simulink model "RightInvariant_EKF"  (R2016b)
settings: Solver=FixedStepDiscrete  StartTime=0.0  StopTime=inf  RelTol=1e-3  EnableMultiTasking=on
InitFcn:
  | RIEKF_InitFcn;
libraries: StateEstimation x3, dspfdesign x2, slrtlib x1, UDP_Communication x1
settings Model: xpc_rtwmakecfg_data=_xpcethercatlib_  ParamWorkspaceSource=ReferencedWorkspace  Creator=robot  LastModifiedBy=Ross Hartley
settings SolverCC: EnableConcurrentExecution=on  ConcurrentTasks=on
settings DataIOCC: SaveFormat=Array  SaveOutput=off  SignalLogging=off  DSMLogging=off  VisualizeSimOutput=off  SaveTime=off
settings OptimizationCC: DefaultParameterBehavior=Inlined  InlineInvariantSignals=on  LifeSpan=inf  SimCompilerOptimization=on  AccelVerboseBuild=on
settings DebuggingCC: AllowSymbolicDim=off  SFUnexpectedBacktrackingDiag=warning  SFNoUnconditionalDefaultTransitionDiag=warning  SFExecutionAtInitializationDiag=none
settings HardwareCC: ProdBitPerPointer=32  ProdBitPerSizeT=32  ProdBitPerPtrDiffT=32  ProdLargestAtomicFloat=None  ProdWordSize=32  ProdLongLongMode=on  ProdHWDeviceType=Generic->32-bit x86 compatible
settings ModelReferenceCC: ParallelModelReferenceMATLABWorkerInit=Copy Base Workspace  ModelReferenceNumInstancesAllowed=Single
settings SFSimCC: SFSimEcho=off
settings SFSimCC: SimUserSources=|
  | p_RightToeBottom_src.c
  | p_LeftToeBottom_src.c
  | J_RightToeBottom_src.c
  | J_LeftToeBottom_src.c
  | p_VectorNav_to_RightToeBottom_src.c
  | R_VectorNav_to_RightToeBottom_src.c
  | p_VectorNav_to_LeftToeBottom_src.c
  | R_VectorNav_to_LeftToeBottom_src.c
  | J_VectorNav_to_RightToeBottom_src.c
  | J_VectorNav_to_LeftToeBottom_src.c
  | p_VectorNav_to_Pelvis_src.c
  | R_VectorNav_to_Pelvis_src.c
  | J_VectorNav_to_Pelvis_src.c
settings SFSimCC: SimUserIncludeDirs=|
  | ..\Cassie_Model\gen\kin\src
  | ..\Cassie_Model\gen\dyn\src
  | \kin\src
settings RTWCC: SystemTargetFile=slrt.tlc  TLCOptions=-axPCMaxOverloads=1000000000 -axPCMaxOverloadLen=1000000000  TemplateMakefile=slrt_default_tmf  Description=Simulink Real-Time  RTWUseSimCustomCode=on  CodeExecutionProfiling=on  RTWCompilerOptimization=on
settings RTWCC: CustomInclude=|
  | ..\Cassie_Model\gen\kin\src
  | ..\Cassie_Model\gen\dyn\src
  | \kin\src
settings RTWCC: CustomSource=|
  | p_RightToeBottom_src.c
  | p_LeftToeBottom_src.c
  | J_RightToeBottom_src.c
  | J_LeftToeBottom_src.c
  | p_VectorNav_to_RightToeBottom_src.c
  | R_VectorNav_to_RightToeBottom_src.c
  | p_VectorNav_to_LeftToeBottom_src.c
  | R_VectorNav_to_LeftToeBottom_src.c
  | J_VectorNav_to_RightToeBottom_src.c
  | J_VectorNav_to_LeftToeBottom_src.c
  | p_VectorNav_to_Pelvis_src.c
  | R_VectorNav_to_Pelvis_src.c
  | J_VectorNav_to_Pelvis_src.c
settings CodeAppCC: GenerateComments=off  MaxIdLength=128  SimulinkBlockComments=off
settings SimulinkRealTimeCC: ExtMode=off
settings ConfigComp: CovMetricSettings=dw  CovHtmlReporting=on  CovSaveCumulativeToWorkspaceVar=on  CovSaveSingleToWorkspaceVar=on  CovExternalEMLEnable=off

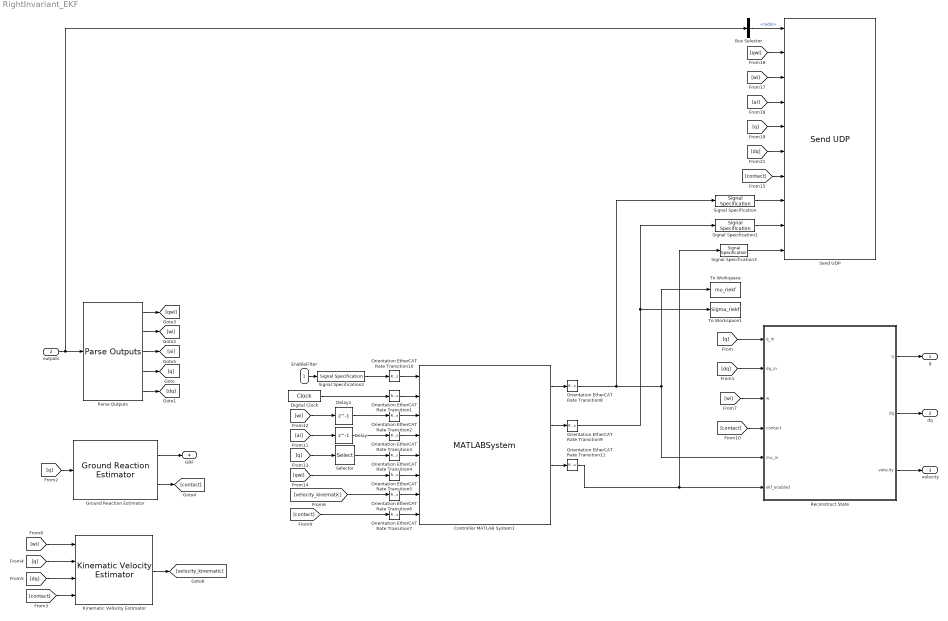
== system RightInvariant_EKF ==
  EnableFilter : Inport
  outputs : Inport  Port=2  OutDataTypeStr=Bus: cassieOutputsBus
  Bus Selector : BusSelector  OutputSignals=radio
  Controller MATLAB System1 : MATLABSystem  System=RIEKF  static_bias_initialization=static_bias_initialization  ekf_update_enabled=ekf_update_enabled  dt=EKF_SampleTime  enable_bias_estimation=enable_bias_estimation  gyro_noise_std=gyro_noise_std  gyro_bias_noise_std=gyro_bias_noise_std  accel_noise_std=accel_noise_std  accel_bias_noise_std=accel_bias_noise_std  contact_noise_std=contact_noise_std  encoder_noise_std=encoder_noise_std  gyro_bias_init=gyro_bias_init  accel_bias_init=accel_bias_init  prior_base_pose_std=prior_base_pose_std  prior_base_velocity_std=prior_base_velocity_std  prior_contact_position_std=prior_contact_position_std  prior_gyro_bias_std=prior_gyro_bias_std  prior_accel_bias_std=prior_accel_bias_std  prior_forward_kinematics_std=prior_forward_kinematics_std  SimulateUsing=Interpreted execution
      mask Type: RIEKF
      mask Display:
      | disp('RIEKF');
      | port_label('input',1,'EnableFilter');
      | port_label('input',2,'t');
      | port_label('input',3,'w');
      | port_label('input',4,'a');
      | port_label('input',5,'e');
      | port_label('input',6,'q_init');
      | port_label('input',7,'v_init');
      | port_label('input',8,'contact');
      | port_label('output',1,'mu');
      | port_label('output',2,'Sigma');
      | port_label('output',3,'enabled');
      | port_label('output',4,'K');
  Delay : Delay  DelayLength=1  InitialCondition=0
  Delay1 : Delay  DelayLength=1  InitialCondition=0
  Digital Clock : DigitalClock  SampleTime=-1
  Ground Reaction Estimator : StateEstimation/Ground Reaction Estimator
  Kinematic Velocity Estimator : StateEstimation/Kinematic Velocity Estimator
  Orientation EtherCAT Rate Transition{1..7,10} (8 alike) : RateTransition  Deterministic=off  OutPortSampleTime=EKF_SampleTime
  Orientation EtherCAT Rate Transition11 : RateTransition  Deterministic=off  OutPortSampleTime=cassieParameters.etherCatSampleTime
  Orientation EtherCAT Rate Transition8 : RateTransition  Deterministic=off  OutPortSampleTime=cassieParameters.etherCatSampleTime
  Orientation EtherCAT Rate Transition9 : RateTransition  Deterministic=off  OutPortSampleTime=cassieParameters.etherCatSampleTime
  Parse Outputs : StateEstimation/Parse Outputs
  Reconstruct State : Subsystem
  Selector : Selector  InputPortWidth=20  IndexOptions=Index vector (dialog)  Indices=[7:20]  OutputSizes=1
  Send UDP : UDP_Communication/Send UDP
  Signal Specification : SignalSpecification  Dimensions=[22,1]
  Signal Specification1 : SignalSpecification  Dimensions=[21,21]
  Signal Specification2 : SignalSpecification  OutDataTypeStr=double  Dimensions=1
  Signal Specification3 : SignalSpecification  Dimensions=1
  To Workspace : ToWorkspace  VariableName=mu_riekf  SaveFormat=Timeseries  SampleTime=-1
  To Workspace1 : ToWorkspace  VariableName=Sigma_riekf  SaveFormat=Timeseries  SampleTime=-1
  q : Outport
  dq : Outport  Port=2
  velocity : Outport  Port=3
  GRF : Outport  Port=4
  wires:
  [velocity_kinematic] -> Orientation EtherCAT Rate Transition6/1
  [qwi] -> Orientation EtherCAT Rate Transition5/1
  Selector/1 -> Orientation EtherCAT Rate Transition4/1
  Delay/1 -> Orientation EtherCAT Rate Transition3/1
  Kinematic Velocity Estimator/1 -> [velocity_kinematic]
  [contact] -> Kinematic Velocity Estimator/4
  [dq] -> Kinematic Velocity Estimator/3
  [q] -> Kinematic Velocity Estimator/2
  [wi] -> Kinematic Velocity Estimator/1
  Ground Reaction Estimator/2 -> [contact]
  Ground Reaction Estimator/1 -> GRF/1
  [q] -> Ground Reaction Estimator/1
  [contact] -> Reconstruct State/4(contact)
  [wi] -> Reconstruct State/3(w)
  Delay1/1 -> Orientation EtherCAT Rate Transition2/1
  Reconstruct State/3(velocity) -> velocity/1
  Reconstruct State/2(dq) -> dq/1
  Reconstruct State/1(q) -> q/1
  [dq] -> Reconstruct State/2(dq_in)
  [q] -> Reconstruct State/1(q_in)
  Parse Outputs/1 -> [qwi]
  Parse Outputs/5 -> [dq]
  Parse Outputs/4 -> [q]
  Parse Outputs/2 -> [wi]
  Parse Outputs/3 -> [ai]
  outputs/1 -> Bus Selector/1, Parse Outputs/1
  [q] -> Selector/1
  [wi] -> Delay1/1
  [ai] -> Delay/1
  [contact] -> Orientation EtherCAT Rate Transition7/1
  EnableFilter/1 -> Signal Specification2/1
  Digital Clock/1 -> Orientation EtherCAT Rate Transition1/1
  Controller MATLAB System1/1 -> Orientation EtherCAT Rate Transition8/1
  Controller MATLAB System1/3 -> Orientation EtherCAT Rate Transition11/1
  Bus Selector/1 -> Send UDP/1  "<radio>"
  [contact] -> Send UDP/7
  [qwi] -> Send UDP/2
  [ai] -> Send UDP/4
  [wi] -> Send UDP/3
  [q] -> Send UDP/5
  [dq] -> Send UDP/6
  Controller MATLAB System1/2 -> Orientation EtherCAT Rate Transition9/1
  Signal Specification/1 -> Send UDP/8
  Signal Specification1/1 -> Send UDP/9
  Signal Specification2/1 -> Orientation EtherCAT Rate Transition10/1
  Signal Specification3/1 -> Send UDP/10
  Orientation EtherCAT Rate Transition10/1 -> Controller MATLAB System1/1
  Orientation EtherCAT Rate Transition1/1 -> Controller MATLAB System1/2
  Orientation EtherCAT Rate Transition2/1 -> Controller MATLAB System1/3
  Orientation EtherCAT Rate Transition3/1 -> Controller MATLAB System1/4
  Orientation EtherCAT Rate Transition4/1 -> Controller MATLAB System1/5
  Orientation EtherCAT Rate Transition5/1 -> Controller MATLAB System1/6
  Orientation EtherCAT Rate Transition6/1 -> Controller MATLAB System1/7
  Orientation EtherCAT Rate Transition7/1 -> Controller MATLAB System1/8
  Orientation EtherCAT Rate Transition8/1 -> Signal Specification/1, To Workspace/1, Reconstruct State/5(mu_in)
  Orientation EtherCAT Rate Transition9/1 -> To Workspace1/1, Signal Specification1/1
  Orientation EtherCAT Rate Transition11/1 -> Signal Specification3/1, Reconstruct State/6(ekf_enabled)

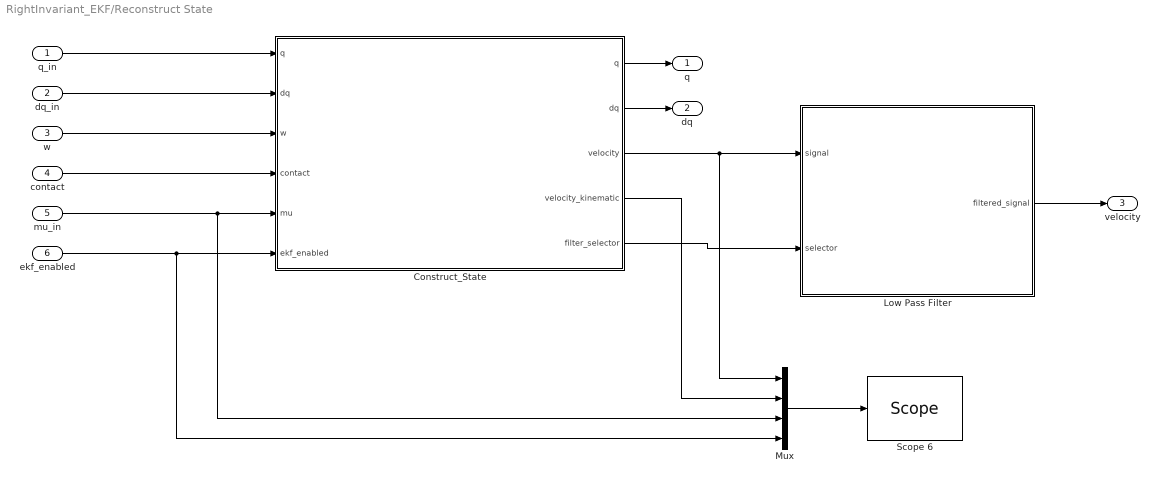
== system RightInvariant_EKF/Reconstruct State ==
  q_in : Inport
  dq_in : Inport  Port=2
  w : Inport  Port=3
  contact : Inport  Port=4
  mu_in : Inport  Port=5
  ekf_enabled : Inport  Port=6
  Construct_State : MATLAB Function  TreatAsAtomicUnit=on
  Low Pass Filter : Subsystem  TreatAsAtomicUnit=on
  Mux : Mux
  Scope 6 : slrtlib/Displays and Logging/Scope   scopeno=2  scopetype=File  autostart=on  viewmode=Numerical  formatstr='%15.6f'  grid=on  ylimits=[0,0]  nosamples=250  noprepostsamples=0  interleave=1  triggermode=FreeRun  triggersignal=1  trigsignalfromport=on  triggerlevel=0.5  triggerslope=Rising  triggerscope=1  triggersample=0  filename=ekf1.dat  mode=Commit  writesize=512  autorestart=on  dynamicfilemode=off  maxwritefilesize=4000*1024^2
  q : Outport
  dq : Outport  Port=2
  velocity : Outport  Port=3
  wires:
  Construct_State/4(velocity_kinematic) -> Mux/2
  contact/1 -> Construct_State/4(contact)
  w/1 -> Construct_State/3(w)
  Construct_State/2(dq) -> dq/1
  ekf_enabled/1 -> Mux/4, Construct_State/6(ekf_enabled)
  q_in/1 -> Construct_State/1("q ")
  Mux/1 -> Scope 6/1
  Construct_State/5(filter_selector) -> Low Pass Filter/2(selector)
  Construct_State/3(velocity) -> Low Pass Filter/1(signal), Mux/1
  Construct_State/1(q) -> q/1
  dq_in/1 -> Construct_State/2("dq ")
  mu_in/1 -> Mux/3, Construct_State/5(mu)
  Low Pass Filter/1(filtered_signal) -> velocity/1

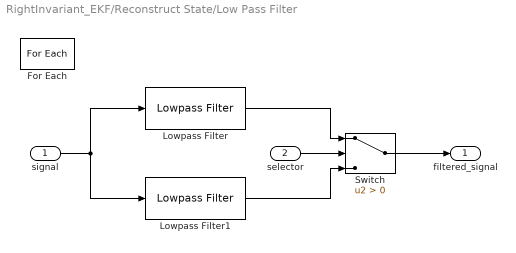
== system RightInvariant_EKF/Reconstruct State/Low Pass Filter ==
  signal : Inport  Partition=on  PartitionDimension=1  PartitionWidth=1
  selector : Inport  Port=2
  For Each : ForEach  DisableCoverage=on  IndexMode=One-based
  Lowpass Filter : dspfdesign/Lowpass Filter  FilterType=FIR  DesignForMinimumOrder=on  FilterOrder=50  PassbandFrequency=1  StopbandFrequency=10  PassbandRipple=1  StopbandAttenuation=20  InheritSampleRate=off  SampleRate=2000  SimulateUsing=Code generation  roundingMode=Floor  coeffsDataTypeStr=fixdt(1,16)
  Lowpass Filter1 : dspfdesign/Lowpass Filter  FilterType=FIR  DesignForMinimumOrder=on  FilterOrder=50  PassbandFrequency=1  StopbandFrequency=5  PassbandRipple=1  StopbandAttenuation=30  InheritSampleRate=off  SampleRate=2000  SimulateUsing=Code generation  roundingMode=Floor  coeffsDataTypeStr=fixdt(1,16)
  Switch : Switch  Criteria=u2 > Threshold
  filtered_signal : Outport  ConcatenationDimension=1
  wires:
  Lowpass Filter1/1 -> Switch/3
  Lowpass Filter/1 -> Switch/1
  Switch/1 -> filtered_signal/1
  selector/1 -> Switch/2
  signal/1 -> Lowpass Filter/1, Lowpass Filter1/1

== matlab function RightInvariant_EKF/Reconstruct State/Construct_State ==
  data: q output; dq output; q input; dq input; w input; contact input; mu input; ekf_enabled input; velocity output; velocity_kinematic output; filter_selector output
function [q, dq, velocity, velocity_kinematic, filter_selector] = Construct_State(q, dq, w, contact, mu, ekf_enabled)
% Construct state vector and body velocity estimate using raw data and ekf
%   
%   Inputs:
%       q           - state position vector
%       dq          - state velocity vector
%       w           - angular velocity, {I}_\omega_{WI}
%       contact     - contact indicator
%       mu          - EKF state estimate
%       ekf_enabled - EKF enable flag
%
%   Outputs:
%       q                   - 
%       dq                  - 
%       velocity            - EKF body velocity, {W}_v_{WB} 
%       velocity_kinematic  - Kinematic body velocity, {B}_v_{WB} 
%       filter_selector     - used to select low pass filter type
%
%
%   Author: Ross Hartley
%   Date:   11/07/2017

%% Settings
use_ekf_position = true;
use_ekf_orientation = false;
use_ekf_velocity = false;

%% Compute kinematic velocity
e = q(7:end);
e_dot = dq(7:end);

if contact(1) == 1
    pL = p_VectorNav_to_LeftToeBottom(e); % {I}_p_{IL}
    J_pL = J_VectorNav_to_LeftToeBottom(e);
    velocity_kinematic = -J_pL(1:3,:)*e_dot - Angles.skew(w)*pL(1:3,:); % {I}_v_{WI}
elseif contact(2) == 1
    pR = p_VectorNav_to_RightToeBottom(e); % {I}_p_{IR}
    J_pR = J_VectorNav_to_RightToeBottom(e);
    velocity_kinematic = -J_pR(1:3,:)*e_dot - Angles.skew(w)*pR(1:3,:); % {I}_v_{WI}
else
    velocity_kinematic = zeros(3,1);
end

%% Reconstruct State
Rbi = R_VectorNav_to_Pelvis(e)';    % R_{BI}

% Position
if use_ekf_position && ekf_enabled
    Rwi = Angles.Quaternion_to_Rotation(mu(7:10))';
    % {W}_p_{WB} =  {W}_p_{WI} +  {W}_p_{IB}
    q(1:3) = mu(1:3) + Rwi * p_VectorNav_to_Pelvis(e); 
end
 
% Orientation
if use_ekf_orientation && ekf_enabled
    Rwi = Angles.Quaternion_to_Rotation(mu(7:10))';
    Rwb = Rwi * Rbi';
    q(4:6) = Angles.Rotation_to_Euler( Rwb );
end

% Velocity
if use_ekf_velocity && ekf_enabled
    Rwi = Angles.Quaternion_to_Rotation(mu(7:10))';
    Rwb = Rwi * Rbi';
    % {W}_v_{WB} =  {W}_v_{WI} + R_{WI} * skew({I}_w_{WI}) * {I}_p_{IB}
    dq(1:3) = mu(4:6) + Rwi * Angles.skew(w) * p_VectorNav_to_Pelvis(e); 
    % {B}_v_{WB} = R_{BW} * {W}_v_{WB}
    velocity = Rwb' * dq(1:3);
    filter_selector = 1;
else
    Rwb = Angles.Euler_to_Rotation(q(4:6));
    Rwi = Rwb * Rbi;
    % {W}_v_{WB} =  R_{WI} * {I}_v_{WI} + R_{WI} * skew({I}_w_{WI}) * {I}_p_{IB}
    dq(1:3) = Rwi * velocity_kinematic + Rwi * Angles.skew(w) * p_VectorNav_to_Pelvis(e); 
    % {B}_v_{WB} = R_{BW} * {W}_v_{WB}
    velocity = Rwb' * dq(1:3);
    filter_selector = 0;
end



end
